simulink model "SteeringWheelSTM32"  (R2024b)
settings: Solver=FixedStepDiscrete  StartTime=0.0  StopTime=1  FixedStep=0.001  RelTol=1e-3  EnableMultiTasking=on
libraries: stm32blockslib x7, simulink x4, stm32h7xxblockslib x1, canmsglib x1, stm32f4xxblockslib x1
settings Model: STM32="{\"DigitalPortRead\":{\"ID\":\"SteeringWheelSTM32:291\"},\"SPIControllerTransfer\":[{\"ID\":\"SteeringWheelSTM32:402\"},{\"ID\":\"SteeringWheelSTM32:417\"},{\"ID\":\"SteeringWheelSTM32:418\"},{\"ID\":\"SteeringWheelSTM32:466\"},{\"ID\":\"SteeringWheelSTM32:471\"},{\"ID\":\"SteeringWheelSTM32:474\"},{\"ID\":\"SteeringWheelSTM32:477\"},{\"ID\":\"SteeringWheelSTM32:480\"}],\"AnalogInputForH7\":{\"ID\":\"SteeringWheelSTM32:529\"}}"  Creator=will  LastModifiedBy=William
settings SolverCC: AlgebraicLoopSolver=TrustRegion
settings DataIOCC: ReturnWorkspaceOutputs=off
settings OptimizationCC: DefaultParameterBehavior=Inlined  EnhancedBackFolding=on  PassReuseOutputArgsAs=Individual arguments  ZeroExternalMemoryAtStartup=off  ZeroInternalMemoryAtStartup=off  MaxStackSize=512  OptimizeBlockOrder=speed  DifferentSizesBufferReuse=on  OptimizationCustomize=off  EfficientTunableParamExpr=on
settings DebuggingCC: ParameterTunabilityLossMsg=error  UnconnectedInputMsg=warning  UnconnectedOutputMsg=warning  UnconnectedLineMsg=warning  ArithmeticOperatorsInVariantConditions=warning
settings HardwareCC: ProdBitPerPointer=32  ProdBitPerSizeT=32  ProdBitPerPtrDiffT=32  ProdLargestAtomicInteger=Long  ProdLargestAtomicFloat=Double  ProdWordSize=32  ProdLongLongMode=on  ProdHWDeviceType=ARM Compatible->ARM Cortex-M
settings ModelReferenceCC: EnableRefExpFcnMdlSchedulingChecks=on
settings SFSimCC: MATLABDynamicMemAlloc=off  CustomCodeUndefinedFunction=UseInterfaceOnly
settings RTWCC: Description=Embedded Coder  SystemTargetFile=ert.tlc  HardwareBoard=STM32H7xx Based (Single-core)  TemplateMakefile=ert_default_tmf  CustomHeaderCode="#include \"stm32h7xx_ll_tim.h\""  CustomInitializer=LL_TIM_EnableCounter(TIM2);  Toolchain=GNU Tools for ARM Embedded Processors  GPUComputeCapability=3.5
settings CodeAppCC: ForceParamTrailComments=on  IgnoreCustomStorageClasses=off  OperatorAnnotations=on  SimulinkDataObjDesc=on  SFDataObjDesc=on  InsertBlockDesc=on
settings ERTTargetCC: TargetLangStandard=C99 (ISO)  CodeReplacementLibrary=ARM Cortex-M  ExtModeTransport=3  ExtModeStaticAlloc=on  ExtModeStaticAllocSize=2048  ExtModeMexFile=ext_xcp  ExtModeIntrfLevel=Level2 - Open

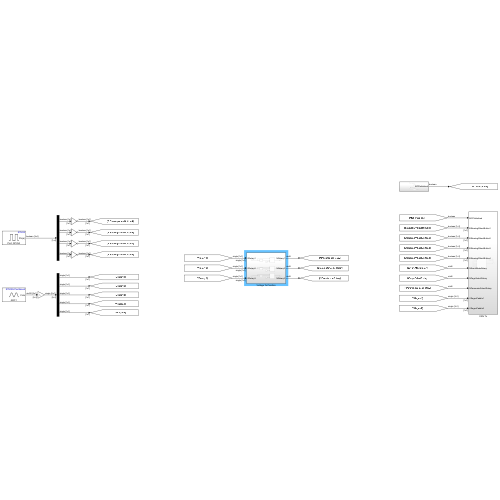
[thumbnail: Simulink's stored preview of the top-level diagram]
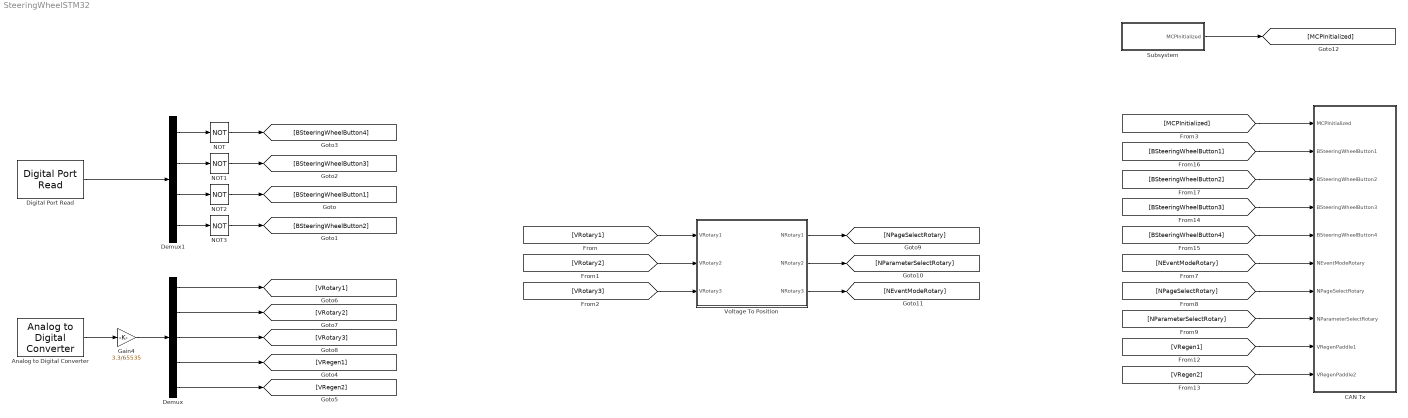
== system SteeringWheelSTM32 ==
  Analog to Digital Converter : stm32h7xxblockslib/Analog to Digital Converter  ADCModule=ADC1  ConversionGroup=Regular  TriggerMode=Read results only  NumberOfConversions=5  EnableBufferConv=on  BufferLength=1  OutputStatus=off  SampleTime=-1  EnableSimPort=off  hoistedMaskSrc=ECSoC/ECSimCodegen/Analog to Digital Converter
  CAN Tx : Subsystem
  Demux : Demux  Outputs=5
  Demux1 : Demux
  Digital Port Read : stm32f4xxblockslib/Digital Port Read  PortName=GPIOA  PinNumber=[9, 10, 11, 12]  ReadOperation=on  IOAsArray=on  SampleTime=-1  EnableSimPort=off  hoistedMaskSrc=ECSoC/ECSimCodegen/Digital Port Read
      settings: LibrarySourceBlock=stm32h7xxblockslib/Digital Port Read
  Gain4 : Gain  Gain=3.3/65535  OutDataTypeStr=single
  NOT{,1..3} (4 alike) : Logic  Operator=NOT  IconShape=distinctive  AllPortsSameDT=off  OutDataTypeStr=boolean
  Subsystem : Subsystem
  Voltage To Position : Subsystem
  wires:
  Demux1/3 -> NOT2/1
  Demux1/4 -> NOT3/1
  Demux1/2 -> NOT1/1
  Demux1/1 -> NOT/1
  [VRotary1] -> Voltage To Position/1(VRotary1)
  [VRotary2] -> Voltage To Position/2(VRotary2)
  [VRotary3] -> Voltage To Position/3(VRotary3)
  Voltage To Position/1(NRotary1) -> [NPageSelectRotary]
  Voltage To Position/2(NRotary2) -> [NParameterSelectRotary]
  Voltage To Position/3(NRotary3) -> [NEventModeRotary]
  [NEventModeRotary] -> CAN Tx/6(NEventModeRotary)
  [NPageSelectRotary] -> CAN Tx/7(NPageSelectRotary)
  [NParameterSelectRotary] -> CAN Tx/8(NParameterSelectRotary)
  [VRegen1] -> CAN Tx/9(VRegenPaddle1)
  [VRegen2] -> CAN Tx/10(VRegenPaddle2)
  [BSteeringWheelButton1] -> CAN Tx/2(BSteeringWheelButton1)
  [BSteeringWheelButton2] -> CAN Tx/3(BSteeringWheelButton2)
  [BSteeringWheelButton3] -> CAN Tx/4(BSteeringWheelButton3)
  [BSteeringWheelButton4] -> CAN Tx/5(BSteeringWheelButton4)
  Digital Port Read/1 -> Demux1/1
  NOT/1 -> [BSteeringWheelButton4]
  NOT1/1 -> [BSteeringWheelButton3]
  NOT2/1 -> [BSteeringWheelButton1]
  NOT3/1 -> [BSteeringWheelButton2]
  Demux/1 -> [VRotary1]
  Demux/2 -> [VRotary2]
  Demux/3 -> [VRotary3]
  Demux/4 -> [VRegen1]
  Demux/5 -> [VRegen2]
  Gain4/1 -> Demux/1
  Analog to Digital Converter/1 -> Gain4/1
  [MCPInitialized] -> CAN Tx/1(MCPInitialized)
  Subsystem/1(MCPInitialized) -> [MCPInitialized]

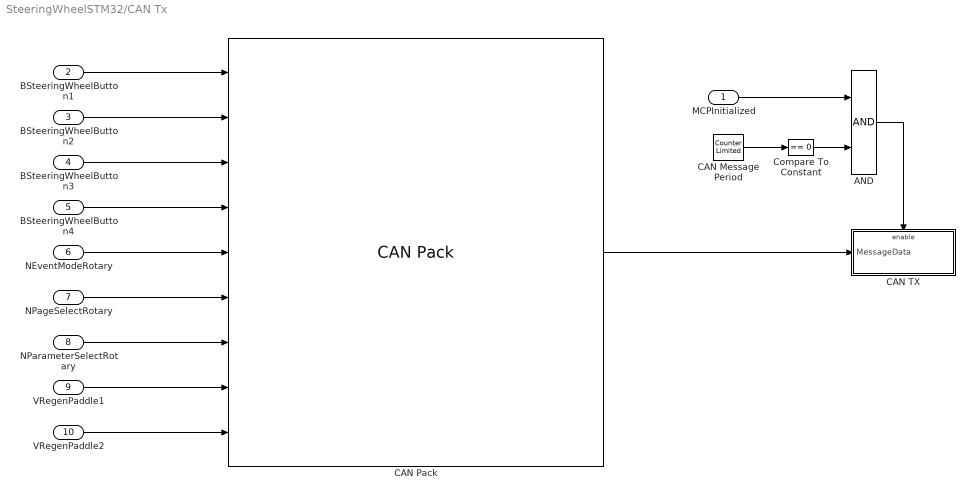
== system SteeringWheelSTM32/CAN Tx ==
  MCPInitialized : Inport
  BSteeringWheelButton1 : Inport  Port=2
  BSteeringWheelButton2 : Inport  Port=3
  BSteeringWheelButton3 : Inport  Port=4
  BSteeringWheelButton4 : Inport  Port=5
  NEventModeRotary : Inport  Port=6
  NPageSelectRotary : Inport  Port=7
  NParameterSelectRotary : Inport  Port=8
  VRegenPaddle1 : Inport  Port=9
  VRegenPaddle2 : Inport  Port=10
  AND : Logic  IconShape=distinctive  AllPortsSameDT=off  OutDataTypeStr=boolean
  CAN Message Period : simulink/Sources/Counter Limited  uplimit=10  tsamp=-1
  CAN Pack : canmsglib/CAN Pack  CANdbFile=C:\Users\William\Downloads\SteeringWheelSTM32\STW_Database.dbc  MsgList=SteeringWheelTest  MsgName=SteeringWheelTest  MsgIDType=Standard (11-bit identifier)  MsgIdentifier=507  CANIDInput=off  MsgLength=6  Remote=off  ApplyMinMax=off  BusOutput=on  SignalInfo={'BSteeringWheelButton1','0','1','LE','unsigned','Standard','0','1','0','0','1';'BSteeringWheelButton2','1','1','LE','unsigned','Standard','0','1','0','0','1';'BSteeringWheelButton3','2','1','LE','unsigned','Standard','0','1','0','0','1';'BSteeringWheelButton4','3','1','LE','unsigned','Standard','0','1','0','0','1';'NEventModeRotary','12','4','LE','unsigned','Standard','0','1','1','1','16';'NPageSelectRotary','4','4','LE','unsigned','Standard','0','1','1','1','16';'NParameterSelectRotary','8','4','LE','unsigned','Standard','0','1','1','1','16';'VRegenPaddle1','16','8','LE','unsigned','Standard','0','0.0129','0','0','3.2895';'VRegenPaddle2','24','8','LE','unsigned','Standard','0','0.0129','0','0','3.2895'}
      settings: LibrarySourceBlock=stmutilitieslib/CAN Pack  DataFormat=CANdb specified signals
  CAN TX : Subsystem  TreatAsAtomicUnit=on
  Compare To Constant : simulink/Logic and Bit Operations/Compare To Constant  relop===  const=0  OutDataTypeStr=boolean
  wires:
  AND/1 -> CAN TX/Enable
  CAN Pack/1 -> CAN TX/1(MessageData)
  CAN Message Period/1 -> Compare To Constant/1
  MCPInitialized/1 -> AND/1
  Compare To Constant/1 -> AND/2
  BSteeringWheelButton1/1 -> CAN Pack/1
  BSteeringWheelButton4/1 -> CAN Pack/4
  BSteeringWheelButton3/1 -> CAN Pack/3
  BSteeringWheelButton2/1 -> CAN Pack/2
  NEventModeRotary/1 -> CAN Pack/5
  NPageSelectRotary/1 -> CAN Pack/6
  NParameterSelectRotary/1 -> CAN Pack/7
  VRegenPaddle1/1 -> CAN Pack/8
  VRegenPaddle2/1 -> CAN Pack/9

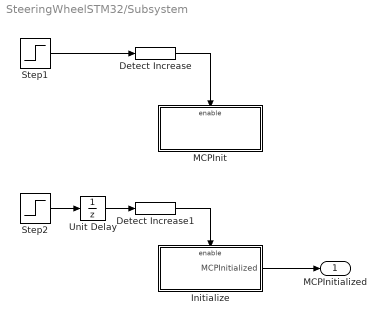
== system SteeringWheelSTM32/Subsystem ==
  Detect Increase : simulink/Logic and Bit Operations/Detect Increase  vinit=0.0  OutDataTypeStr=boolean
  Detect Increase1 : simulink/Logic and Bit Operations/Detect Increase  vinit=0.0  OutDataTypeStr=boolean
  Initialize : Subsystem  TreatAsAtomicUnit=on
  MCPInit : Subsystem  TreatAsAtomicUnit=on
  Step1 : Step
  Step2 : Step
  Unit Delay : UnitDelay  SampleTime=-1  HasFrameUpgradeWarning=on
  MCPInitialized : Outport
  wires:
  Step1/1 -> Detect Increase/1
  Unit Delay/1 -> Detect Increase1/1
  Detect Increase1/1 -> Initialize/Enable
  Detect Increase/1 -> MCPInit/Enable
  Step2/1 -> Unit Delay/1
  Initialize/1(MCPInitialized) -> MCPInitialized/1

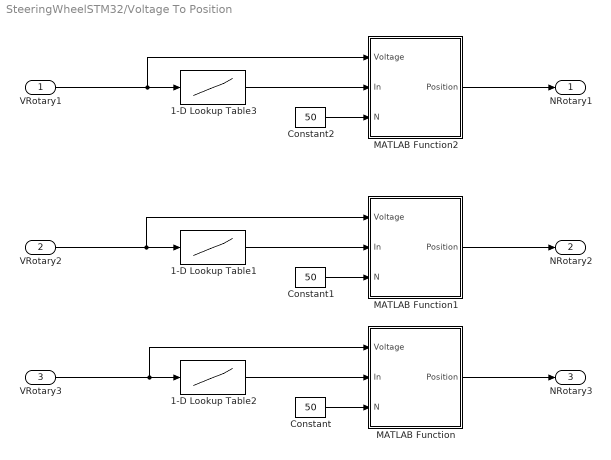
== system SteeringWheelSTM32/Voltage To Position ==
  VRotary1 : Inport  OutDataTypeStr=single
  VRotary2 : Inport  Port=2  OutDataTypeStr=single
  VRotary3 : Inport  Port=3  OutDataTypeStr=single
  1-D Lookup Table1 : Lookup_n-D  NumberOfTableDimensions=1  BreakpointsForDimension1=[0.38, 0.58, 0.78, 0.97, 1.16, 1.35, 1.53, 1.73, 1.90, 2.08, 2.27, 2.44, 2.62, 2.80, 2.97, 3.14]  Table=[1, 16, 15, 14, 13, 12, 11, 10, 9, 8, 7, 6, 5, 4, 3, 2]  InterpMethod=Nearest  InternalRulePriority=Speed  OutDataTypeStr=uint8  RndMeth=Simplest
  1-D Lookup Table2 : Lookup_n-D  NumberOfTableDimensions=1  BreakpointsForDimension1=[0.38, 0.58, 0.78, 0.97, 1.16, 1.35, 1.53, 1.73, 1.90, 2.08, 2.27, 2.44, 2.62, 2.80, 2.97, 3.14]  Table=[1, 16, 15, 14, 13, 12, 11, 10, 9, 8, 7, 6, 5, 4, 3, 2]  InterpMethod=Nearest  InternalRulePriority=Speed  OutDataTypeStr=uint8  RndMeth=Simplest
  1-D Lookup Table3 : Lookup_n-D  NumberOfTableDimensions=1  BreakpointsForDimension1=[0.38, 0.58, 0.78, 0.97, 1.16, 1.35, 1.53, 1.73, 1.90, 2.08, 2.27, 2.44, 2.62, 2.80, 2.97, 3.14]  Table=[1, 16, 15, 14, 13, 12, 11, 10, 9, 8, 7, 6, 5, 4, 3, 2]  InterpMethod=Nearest  InternalRulePriority=Speed  OutDataTypeStr=uint8  RndMeth=Simplest
  Constant : Constant  Value=50
  Constant1 : Constant  Value=50
  Constant2 : Constant  Value=50
  MATLAB Function : MATLAB Function  TreatAsAtomicUnit=on
  MATLAB Function1 : MATLAB Function  TreatAsAtomicUnit=on
  MATLAB Function2 : MATLAB Function  TreatAsAtomicUnit=on
  NRotary1 : Outport  OutDataTypeStr=uint8
  NRotary2 : Outport  Port=2  OutDataTypeStr=uint8
  NRotary3 : Outport  Port=3  OutDataTypeStr=uint8
  wires:
  VRotary3/1 -> MATLAB Function/1(Voltage), 1-D Lookup Table2/1
  Constant/1 -> MATLAB Function/3(N)
  MATLAB Function/1(Position) -> NRotary3/1
  MATLAB Function1/1(Position) -> NRotary2/1
  VRotary2/1 -> MATLAB Function1/1(Voltage), 1-D Lookup Table1/1
  Constant1/1 -> MATLAB Function1/3(N)
  1-D Lookup Table1/1 -> MATLAB Function1/2(In)
  MATLAB Function2/1(Position) -> NRotary1/1
  VRotary1/1 -> MATLAB Function2/1(Voltage), 1-D Lookup Table3/1
  Constant2/1 -> MATLAB Function2/3(N)
  1-D Lookup Table3/1 -> MATLAB Function2/2(In)
  1-D Lookup Table2/1 -> MATLAB Function/2(In)

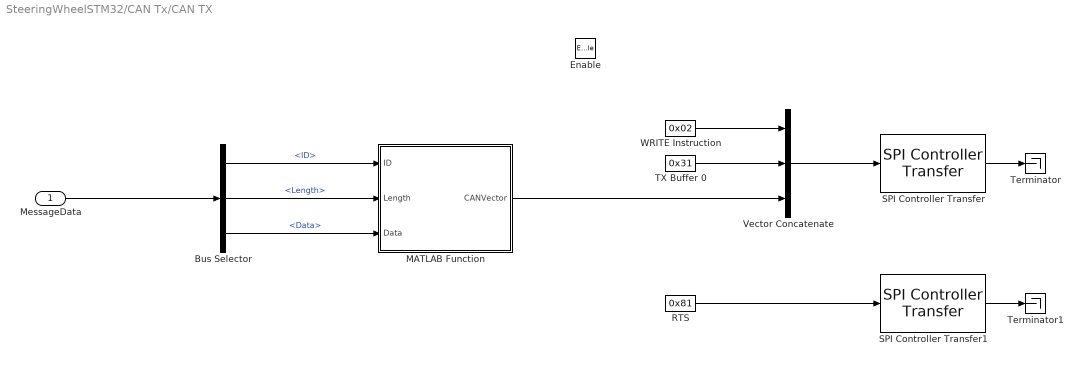
== system SteeringWheelSTM32/CAN Tx/CAN TX ==
  MessageData : Inport
  Enable : EnablePort
  Bus Selector : BusSelector  OutputSignals=ID,Length,Data
  MATLAB Function : MATLAB Function  TreatAsAtomicUnit=on
  RTS : Constant  Value=0x81  OutDataTypeStr=uint8  SampleTime=-1
  SPI Controller Transfer : stm32blockslib/SPI Controller Transfer  Priority=1  SPIModuleSelect=SPI1  ClockPolarity=Low  ClockPhase=1 Edge  SPIModule=uint32(0)  Mode=Master  BusSpeed=uint32(1000000)  FirstBitToTransfer=Most significant bit (MSB)  ClockMode=0  BlockFunction=Transfer  EnableRegisterAddress=off  RegisterAddress=0  OutputDataType=uint8  OutputDataLength=1  OutputStatus=off  BlockingMode=on  Timeout=0.01  DataBits=8  UseCustomSSPin=Explicit GPIO calls  ActiveLowSSPin=Active low  Port_Select=GPIOA  Pin=4
      settings: LibrarySourceBlock=stm32h7xxblockslib/SPI Controller Transfer
  SPI Controller Transfer1 : stm32blockslib/SPI Controller Transfer  Priority=5  SPIModuleSelect=SPI1  ClockPolarity=Low  ClockPhase=1 Edge  SPIModule=uint32(0)  Mode=Master  BusSpeed=uint32(1000000)  FirstBitToTransfer=Most significant bit (MSB)  ClockMode=0  BlockFunction=Transfer  EnableRegisterAddress=off  RegisterAddress=0  OutputDataType=uint8  OutputDataLength=1  OutputStatus=off  BlockingMode=on  Timeout=0.01  DataBits=8  UseCustomSSPin=Explicit GPIO calls  ActiveLowSSPin=Active low  Port_Select=GPIOA  Pin=4
      settings: LibrarySourceBlock=stm32h7xxblockslib/SPI Controller Transfer
  TX Buffer 0 : Constant  Value=0x31  OutDataTypeStr=uint8  SampleTime=-1
  Terminator : Terminator
  Terminator1 : Terminator
  Vector Concatenate : Concatenate  NumInputs=3
  WRITE Instruction : Constant  Value=0x02  OutDataTypeStr=uint8  SampleTime=-1
  wires:
  SPI Controller Transfer1/1 -> Terminator1/1
  Bus Selector/2 -> MATLAB Function/2(Length)  "<Length>"
  Bus Selector/1 -> MATLAB Function/1(ID)  "<ID>"
  MATLAB Function/1(CANVector) -> Vector Concatenate/3
  TX Buffer 0/1 -> Vector Concatenate/2
  Bus Selector/3 -> MATLAB Function/3(Data)  "<Data>"
  MessageData/1 -> Bus Selector/1
  WRITE Instruction/1 -> Vector Concatenate/1
  SPI Controller Transfer/1 -> Terminator/1
  Vector Concatenate/1 -> SPI Controller Transfer/1
  RTS/1 -> SPI Controller Transfer1/1

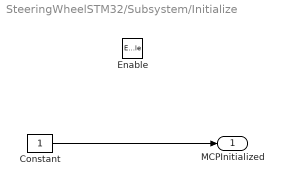
== system SteeringWheelSTM32/Subsystem/Initialize ==
  Enable : EnablePort
  Constant : Constant  OutDataTypeStr=boolean
  MCPInitialized : Outport
  wires:
  Constant/1 -> MCPInitialized/1

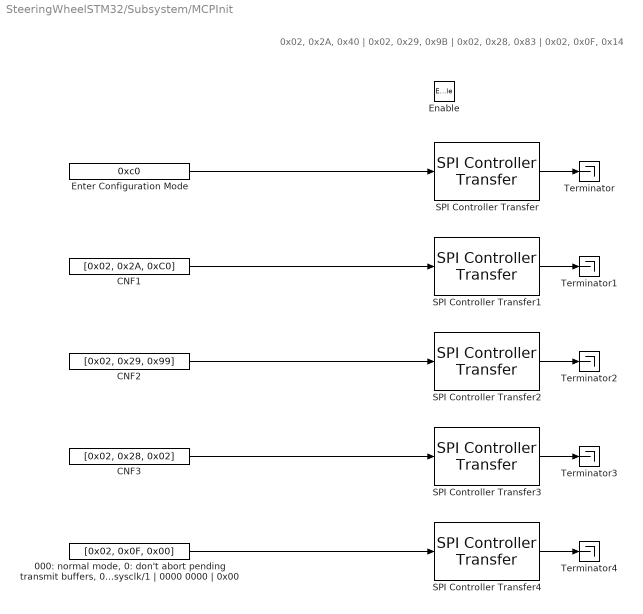
== system SteeringWheelSTM32/Subsystem/MCPInit ==
  note: 0x02, 0x2A, 0x40 | 0x02, 0x29, 0x9B | 0x02, 0x28, 0x83 | 0x02, 0x0F, 0x14
  Enable : EnablePort
  " 000: normal mode, 0: don't abort pending transmit buffers, 0: one-shot disabled, 0: CLKOUT disabled, 00: sysclk/1 | 0000 0000 | 0x00" : Constant  Value=[0x02, 0x0F, 0x00]  OutDataTypeStr=uint8
  CNF1 : Constant  Value=[0x02, 0x2A, 0xC0]  OutDataTypeStr=uint8
  CNF2 : Constant  Value=[0x02, 0x29, 0x99]  OutDataTypeStr=uint8
  CNF3 : Constant  Value=[0x02, 0x28, 0x02]  OutDataTypeStr=uint8
  Enter Configuration Mode : Constant  Value=0xc0  OutDataTypeStr=uint8
  SPI Controller Transfer : stm32blockslib/SPI Controller Transfer  Priority=4  SPIModuleSelect=SPI1  ClockPolarity=Low  ClockPhase=1 Edge  SPIModule=uint32(0)  Mode=Master  BusSpeed=uint32(1000000)  FirstBitToTransfer=Most significant bit (MSB)  ClockMode=0  BlockFunction=Transfer  EnableRegisterAddress=off  RegisterAddress=0  OutputDataType=uint8  OutputDataLength=1  OutputStatus=off  BlockingMode=on  Timeout=0.01  DataBits=8  UseCustomSSPin=Explicit GPIO calls  ActiveLowSSPin=Active low  Port_Select=GPIOA  Pin=4
      settings: LibrarySourceBlock=stm32h7xxblockslib/SPI Controller Transfer
  SPI Controller Transfer1 : stm32blockslib/SPI Controller Transfer  Priority=5  SPIModuleSelect=SPI1  ClockPolarity=Low  ClockPhase=1 Edge  SPIModule=uint32(0)  Mode=Master  BusSpeed=uint32(1000000)  FirstBitToTransfer=Most significant bit (MSB)  ClockMode=0  BlockFunction=Transfer  EnableRegisterAddress=off  RegisterAddress=0  OutputDataType=uint8  OutputDataLength=1  OutputStatus=off  BlockingMode=on  Timeout=0.01  DataBits=8  UseCustomSSPin=Explicit GPIO calls  ActiveLowSSPin=Active low  Port_Select=GPIOA  Pin=4
      settings: LibrarySourceBlock=stm32h7xxblockslib/SPI Controller Transfer
  SPI Controller Transfer2 : stm32blockslib/SPI Controller Transfer  Priority=6  SPIModuleSelect=SPI1  ClockPolarity=Low  ClockPhase=1 Edge  SPIModule=uint32(0)  Mode=Master  BusSpeed=uint32(1000000)  FirstBitToTransfer=Most significant bit (MSB)  ClockMode=0  BlockFunction=Transfer  EnableRegisterAddress=off  RegisterAddress=0  OutputDataType=uint8  OutputDataLength=1  OutputStatus=off  BlockingMode=on  Timeout=0.01  DataBits=8  UseCustomSSPin=Explicit GPIO calls  ActiveLowSSPin=Active low  Port_Select=GPIOA  Pin=4
      settings: LibrarySourceBlock=stm32h7xxblockslib/SPI Controller Transfer
  SPI Controller Transfer3 : stm32blockslib/SPI Controller Transfer  Priority=7  SPIModuleSelect=SPI1  ClockPolarity=Low  ClockPhase=1 Edge  SPIModule=uint32(0)  Mode=Master  BusSpeed=uint32(1000000)  FirstBitToTransfer=Most significant bit (MSB)  ClockMode=0  BlockFunction=Transfer  EnableRegisterAddress=off  RegisterAddress=0  OutputDataType=uint8  OutputDataLength=1  OutputStatus=off  BlockingMode=on  Timeout=0.01  DataBits=8  UseCustomSSPin=Explicit GPIO calls  ActiveLowSSPin=Active low  Port_Select=GPIOA  Pin=4
      settings: LibrarySourceBlock=stm32h7xxblockslib/SPI Controller Transfer
  SPI Controller Transfer4 : stm32blockslib/SPI Controller Transfer  Priority=8  SPIModuleSelect=SPI1  ClockPolarity=Low  ClockPhase=1 Edge  SPIModule=uint32(0)  Mode=Master  BusSpeed=uint32(1000000)  FirstBitToTransfer=Most significant bit (MSB)  ClockMode=0  BlockFunction=Transfer  EnableRegisterAddress=off  RegisterAddress=0  OutputDataType=uint8  OutputDataLength=1  OutputStatus=off  BlockingMode=on  Timeout=0.01  DataBits=8  UseCustomSSPin=Explicit GPIO calls  ActiveLowSSPin=Active low  Port_Select=GPIOA  Pin=4
      settings: LibrarySourceBlock=stm32h7xxblockslib/SPI Controller Transfer
  Terminator{,1..4} (5 alike) : Terminator
  wires:
  SPI Controller Transfer/1 -> Terminator/1
  Enter Configuration Mode/1 -> SPI Controller Transfer/1
  CNF1/1 -> SPI Controller Transfer1/1
  SPI Controller Transfer1/1 -> Terminator1/1
  CNF2/1 -> SPI Controller Transfer2/1
  SPI Controller Transfer2/1 -> Terminator2/1
  CNF3/1 -> SPI Controller Transfer3/1
  SPI Controller Transfer3/1 -> Terminator3/1
  " 000: normal mode, 0: don't abort pending transmit buffers, 0: one-shot disabled, 0: CLKOUT disabled, 00: sysclk/1 | 0000 0000 | 0x00"/1 -> SPI Controller Transfer4/1
  SPI Controller Transfer4/1 -> Terminator4/1

== matlab function SteeringWheelSTM32/CAN Tx/CAN TX/MATLAB Function ==
  data: ID input uint32; CANVector output uint8; Length input uint8; Data input uint8
function CANVector = ConvertToVector(ID, Length, Data)
    %#codegen
    id_u16 = uint16(ID);
    len_u8 = uint8(Length);

    CANVector = zeros(1, 13, 'uint8');  % 13 bytes only — no instruction

    CANVector(1) = uint8(bitshift(id_u16, -3));              % SIDH: ID[10:3]
    CANVector(2) = uint8(bitshift(bitand(id_u16, uint16(7)), 5)); % SIDL: ID[2:0]<<5, EXIDE=0
    CANVector(3) = uint8(0);   % EID8 unused
    CANVector(4) = uint8(0);   % EID0 unused
    CANVector(5) = bitand(len_u8, uint8(15));  % DLC
    for i = 1:8
        CANVector(5+i) = uint8(Data(i));
    end

== matlab function SteeringWheelSTM32/Voltage To Position/MATLAB Function ==
  data: Voltage input; In input; Position output; N input
function Position = Debounce(Voltage, In, N)
    persistent current candidate count;
    
    if isempty(current)
        current = In;
        candidate = In;
        count = 0;
    end
    
    % IGNORE reading entirely if voltage is near 0 (in transition)
    if Voltage < 0.15
        Position = current;  % just hold, don't even consider updating
        return;
    end
    
    if In == candidate
        count = count + 1;
    else
        candidate = In;
        count = 0;
    end
    
    if count >= N
        current = candidate;
    end
    
    Position = current;
end

== matlab function SteeringWheelSTM32/Voltage To Position/MATLAB Function1 ==
  data: Voltage input; In input; Position output; N input
function Position = Debounce(Voltage, In, N)
    persistent current candidate count;
    
    if isempty(current)
        current = In;
        candidate = In;
        count = 0;
    end
    
    % IGNORE reading entirely if voltage is near 0 (in transition)
    if Voltage < 0.15
        Position = current;  % just hold, don't even consider updating
        return;
    end
    
    if In == candidate
        count = count + 1;
    else
        candidate = In;
        count = 0;
    end
    
    if count >= N
        current = candidate;
    end
    
    Position = current;
end

== matlab function SteeringWheelSTM32/Voltage To Position/MATLAB Function2 ==
  data: Voltage input; In input; Position output; N input
function Position = Debounce(Voltage, In, N)
    persistent current candidate count;
    
    if isempty(current)
        current = In;
        candidate = In;
        count = 0;
    end
    
    % IGNORE reading entirely if voltage is near 0 (in transition)
    if Voltage < 0.15
        Position = current;  % just hold, don't even consider updating
        return;
    end
    
    if In == candidate
        count = count + 1;
    else
        candidate = In;
        count = 0;
    end
    
    if count >= N
        current = candidate;
    end
    
    Position = current;
end
